simulink model "TwoTank_LQ"  (R2022b)
settings: Solver=VariableStepAuto  StartTime=0.0  StopTime=2500  RelTol=1e-3
values from neighbouring files (symbols this model uses):
  g = 9.81    [compute_equilibrium.m]    (also in main_LQ.m)
  h2_bar = (a1 / (S1 * k))^2 * h1_ref    [compute_equilibrium.m]    (also in main_LQ.m = x_bar(2))
  K_lq = lqr(A_lin, B_lin, Q, R)    [main_LQ.m]
  q_bar = u_bar    [main_LQ.m]
settings Model: Creator=fabio  LastModifiedBy=marco
settings SolverCC: AlgebraicLoopSolver=TrustRegion
settings OptimizationCC: BlockReduction=off  DefaultParameterBehavior=Inlined  BufferReuse=off
settings DebuggingCC: UnconnectedInputMsg=warning  UnconnectedOutputMsg=warning  UnconnectedLineMsg=warning  SFMachineParentedDataDiag=warning
settings ModelReferenceCC: EnableRefExpFcnMdlSchedulingChecks=on
settings RTWCC: DLArmComputeVersion=19.05

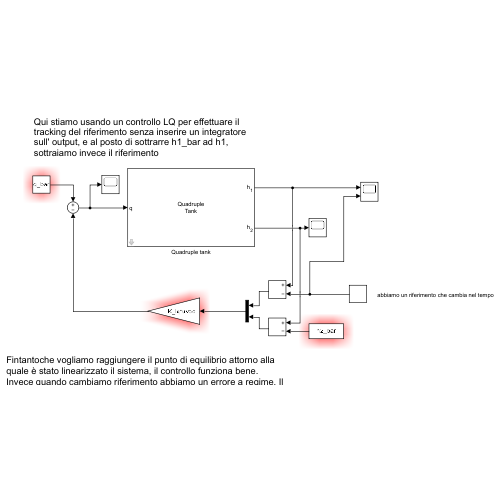
[thumbnail: Simulink's stored preview of the top-level diagram]
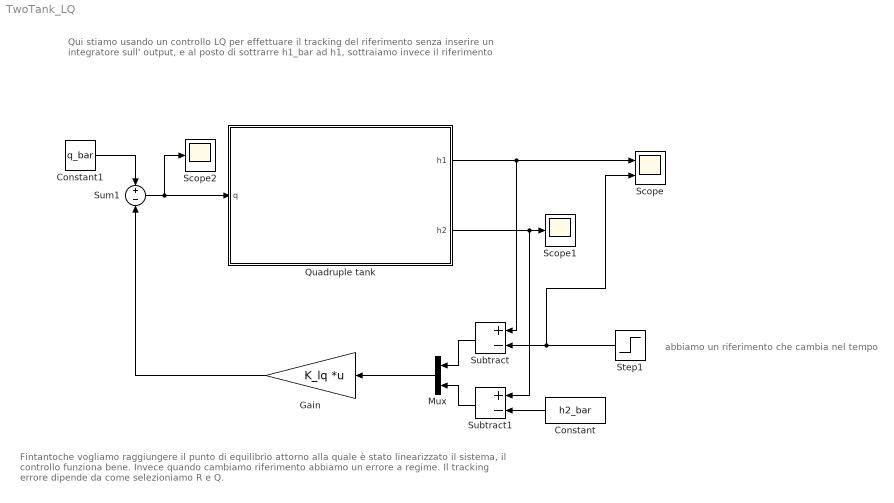
== system TwoTank_LQ ==
  note: Fintantoche vogliamo raggiungere il punto di equilibrio attorno alla quale è stato linearizzato il sistema, il controllo funziona bene.
      | Invece quando cambiamo riferimento abbiamo un errore a regime. Il tracking errore dipende da come selezioniamo R e Q.
  note: abbiamo un riferimento che cambia nel tempo
  note: Qui stiamo usando un controllo LQ per effettuare il tracking del riferimento senza inserire un integratore sull' output, e al posto di sottrarre h1_bar ad h1, sottraiamo invece il riferimento
  Constant : Constant  Value=h2_bar
  Constant1 : Constant  Value=q_bar
  Gain : Gain  Gain=K_lq  Multiplication=Matrix(K*u) (u vector)
  Mux : Mux  Inputs=2
  Quadruple tank : Subsystem  mask{h_0=[ 0.5; 0.2], At=[1.31e-4, 9.27e-5], S=[0.06, 0.06], gamma=0.4, enable_saturation=on, enable_rate=off}
      mask prompts: h_0 "Initial level"; At "Tank discharge constant"; S "Tank section"; gamma "Valve split coefficient"; enable_saturation "Control saturation"; enable_rate "Control rate limit"
      mask DialogControl h_0 Tooltip: [cm]
      mask DialogControl At Tooltip: [cm^2]
      mask DialogControl S Tooltip: [cm^2]
      mask DialogControl gamma Tooltip: [cm/s^2]
      mask Display:
      | disp('Quadruple\nTank');
      | port_label('input', 1, 'q', 'interpreter', 'tex');
      | port_label('output', 1, 'h_1', 'interpreter', 'tex');
      | port_label('output', 2, 'h_2', 'interpreter', 'tex');
  Scope : Scope  NumInputPorts=2
  Scope1 : Scope
  Scope2 : Scope
  Step1 : Step  Time=1000  Before=0.8  After=1.25  SampleTime=0
  Subtract : Sum  Inputs=+-
  Subtract1 : Sum  Inputs=+-
  Sum1 : Sum  Inputs=+|-
  wires:
  Quadruple tank/1(h1) -> Subtract/1, Scope/1
  Quadruple tank/2(h2) -> Subtract1/1, Scope1/1
  Sum1/1 -> Quadruple tank/1(q), Scope2/1
  Step1/1 -> Scope/2, Subtract/2
  Subtract/1 -> Mux/1
  Mux/1 -> Gain/1
  Gain/1 -> Sum1/2
  Constant1/1 -> Sum1/1
  Subtract1/1 -> Mux/2
  Constant/1 -> Subtract1/2

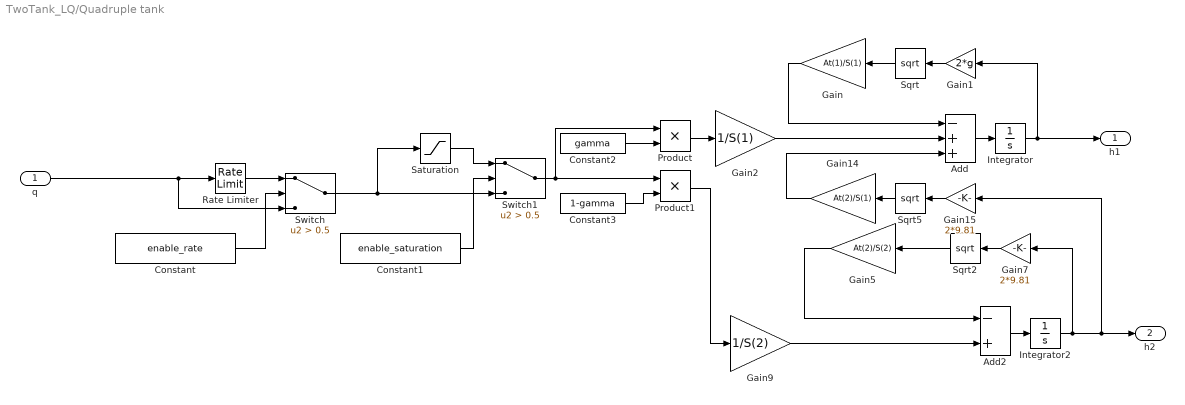
== system TwoTank_LQ/Quadruple tank ==
  q : Inport
  Add : Sum  Inputs=-++
  Add2 : Sum  Inputs=-+
  Constant : Constant  Value=enable_rate
  Constant1 : Constant  Value=enable_saturation
  Constant2 : Constant  Value=gamma
  Constant3 : Constant  Value=1-gamma
  Gain : Gain  Gain=At(1)/S(1)
  Gain1 : Gain  Gain=2*g
  Gain14 : Gain  Gain=At(2)/S(1)
  Gain15 : Gain  Gain=2*9.81
  Gain2 : Gain  Gain=1/S(1)
  Gain5 : Gain  Gain=At(2)/S(2)
  Gain7 : Gain  Gain=2*9.81
  Gain9 : Gain  Gain=1/S(2)
  Integrator : Integrator  InitialCondition=h_0(1)  LimitOutput=on  UpperSaturationLimit=1.3  LowerSaturationLimit=0
  Integrator2 : Integrator  InitialCondition=h_0(2)  LimitOutput=on  UpperSaturationLimit=1.2  LowerSaturationLimit=0
  Product : Product
  Product1 : Product
  Rate Limiter : RateLimiter  SampleTimeMode=inherited  LinearizeAsGain=off
  Saturation : Saturate  UpperLimit=1e-3  LowerLimit=1e-4  LinearizeAsGain=off
  Sqrt : Sqrt
  Sqrt2 : Sqrt
  Sqrt5 : Sqrt
  Switch : Switch  Criteria=u2 > Threshold  Threshold=0.5  SaturateOnIntegerOverflow=off  InputSameDT=off
  Switch1 : Switch  Criteria=u2 > Threshold  Threshold=0.5  SaturateOnIntegerOverflow=off  InputSameDT=off
  h1 : Outport
  h2 : Outport  Port=2
  wires:
  Integrator/1 -> Gain1/1, h1/1
  Add/1 -> Integrator/1
  Gain1/1 -> Sqrt/1
  Sqrt/1 -> Gain/1
  Gain/1 -> Add/1
  Gain2/1 -> Add/2
  Product/1 -> Gain2/1
  Add2/1 -> Integrator2/1
  Gain7/1 -> Sqrt2/1
  Sqrt2/1 -> Gain5/1
  Gain9/1 -> Add2/2
  Product1/1 -> Gain9/1
  Gain15/1 -> Sqrt5/1
  Sqrt5/1 -> Gain14/1
  Integrator2/1 -> Gain7/1, Gain15/1, h2/1
  Gain14/1 -> Add/3
  Gain5/1 -> Add2/1
  Constant2/1 -> Product/2
  Constant3/1 -> Product1/2
  Rate Limiter/1 -> Switch/1
  q/1 -> Switch/3, Rate Limiter/1
  Constant/1 -> Switch/2
  Saturation/1 -> Switch1/1
  Switch/1 -> Saturation/1, Switch1/3
  Constant1/1 -> Switch1/2
  Switch1/1 -> Product1/1, Product/1
